simulink model "EV_HW"  (R2025b)
settings: Solver=VariableStepAuto  StartTime=0.0  StopTime=20  RelTol=1e-3
settings Model: Creator=USER  LastModifiedBy=USER

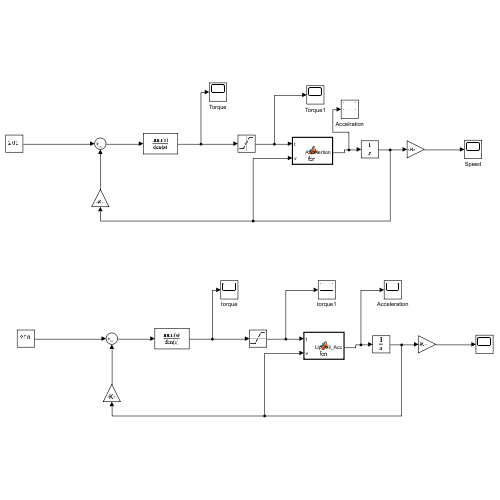
[thumbnail: Simulink's stored preview of the top-level diagram]
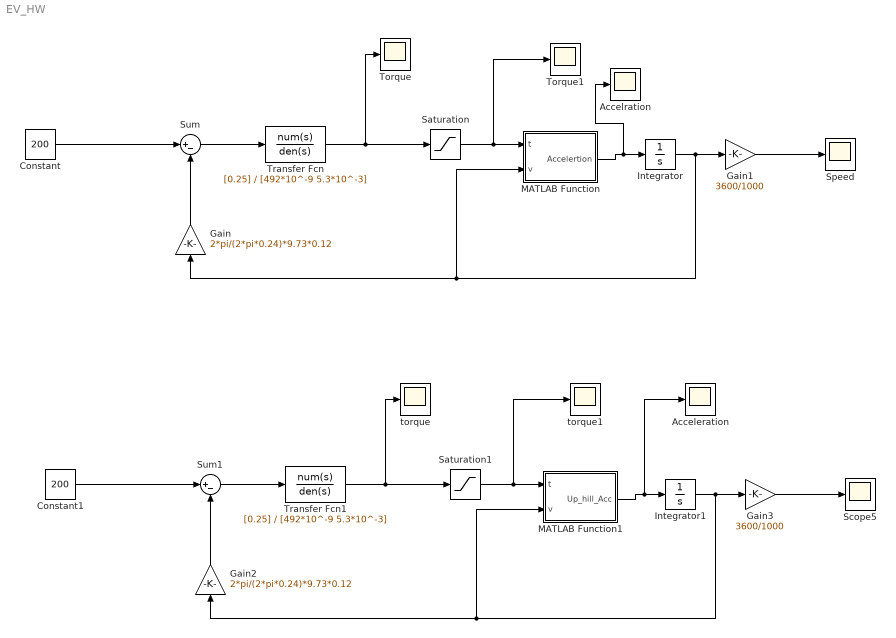
== system EV_HW ==
  Acceleration : Scope
      settings: ActiveDisplayYMinimum=-3.71417558600231  ActiveDisplayYMaximum=9.72039667717068  DataLoggingVariableName=ScopeData7
  Accelration : Scope
      settings: ActiveDisplayYMinimum=-1.061924810246671  ActiveDisplayYMaximum=7.5981202561669088  DataLoggingVariableName=ScopeData6
  Constant : Constant  Value=200
  Constant1 : Constant  Value=200
  Gain : Gain  Gain=2*pi/(2*pi*0.24)*9.73*0.12
  Gain1 : Gain  Gain=3600/1000
  Gain2 : Gain  Gain=2*pi/(2*pi*0.24)*9.73*0.12
  Gain3 : Gain  Gain=3600/1000
  Integrator : Integrator
  Integrator1 : Integrator
  MATLAB Function : MATLAB Function  TreatAsAtomicUnit=on
  MATLAB Function1 : MATLAB Function  TreatAsAtomicUnit=on
  Saturation : Saturate  UpperLimit=601  LowerLimit=0
  Saturation1 : Saturate  UpperLimit=601  LowerLimit=0
  Scope5 : Scope
      settings: ActiveDisplayYMinimum=-110.56280077445663  ActiveDisplayYMaximum=288.91785013295316  DataLoggingVariableName=ScopeData5
  Speed : Scope
      settings: ActiveDisplayYMinimum=98.528705947873661  ActiveDisplayYMaximum=146.88040102580919  DataLoggingVariableName=ScopeData2
  Sum : Sum  Inputs=|+-
  Sum1 : Sum  Inputs=|+-
  Torque : Scope
      settings: ActiveDisplayYMinimum=-1178.9496180143742  ActiveDisplayYMaximum=10610.54656212937
  Torque1 : Scope
      settings: ActiveDisplayYMinimum=-75.124999999999986  ActiveDisplayYMaximum=676.125
  Transfer Fcn : TransferFcn  Numerator=[0.25]  Denominator=[492*10^-9 5.3*10^-3]
  Transfer Fcn1 : TransferFcn  Numerator=[0.25]  Denominator=[492*10^-9 5.3*10^-3]
  torque : Scope
      settings: ActiveDisplayYMinimum=-1178.9709330523028  ActiveDisplayYMaximum=10610.738397470728  DataLoggingVariableName=ScopeData3
  torque1 : Scope
      settings: ActiveDisplayYMinimum=-75.124999999999986  ActiveDisplayYMaximum=676.125  DataLoggingVariableName=ScopeData4
  wires:
  Constant/1 -> Sum/1
  Gain/1 -> Sum/2
  Sum/1 -> Transfer Fcn/1
  Transfer Fcn/1 -> Torque/1, Saturation/1
  Saturation/1 -> Torque1/1, MATLAB Function/1(t)
  MATLAB Function/1(Accelertion) -> Accelration/1, Integrator/1
  Integrator/1 -> MATLAB Function/2(v), Gain/1, Gain1/1
  Gain1/1 -> Speed/1
  Saturation1/1 -> torque1/1, MATLAB Function1/1(t)
  Gain3/1 -> Scope5/1
  Integrator1/1 -> MATLAB Function1/2(v), Gain2/1, Gain3/1
  MATLAB Function1/1(Up_hill_Acc) -> Acceleration/1, Integrator1/1
  Sum1/1 -> Transfer Fcn1/1
  Transfer Fcn1/1 -> torque/1, Saturation1/1
  Gain2/1 -> Sum1/2
  Constant1/1 -> Sum1/1

== matlab function EV_HW/MATLAB Function1 ==
  data: t input; Up_hill_Acc output; v input
function Up_hill_Acc = fcn(t, v)

Up_hill_Acc = (0.6*40.5*t-413-0.3381*v^2-2108*sind(45)*9.81)/2108;

end

== matlab function EV_HW/MATLAB Function ==
  data: t input; Accelertion output; v input
function Accelertion = fcn(t, v)

Accelertion = (0.6*40.5*t-413-0.3381*v^2)/2108;

end
